simulink model "modello_assex"  (R2021a)
settings: Solver=VariableStepAuto  StartTime=0.0  StopTime=0.2  RelTol=1e-3
InitFcn:
  | global par;
  | 
  | par = parametri();
undefined symbols (not defined in the file or in its folder): accelerazioni
settings Model: Creator=user  LastModifiedBy=stefa
settings SolverCC: AlgebraicLoopSolver=TrustRegion
settings DebuggingCC: SFMachineParentedDataDiag=warning

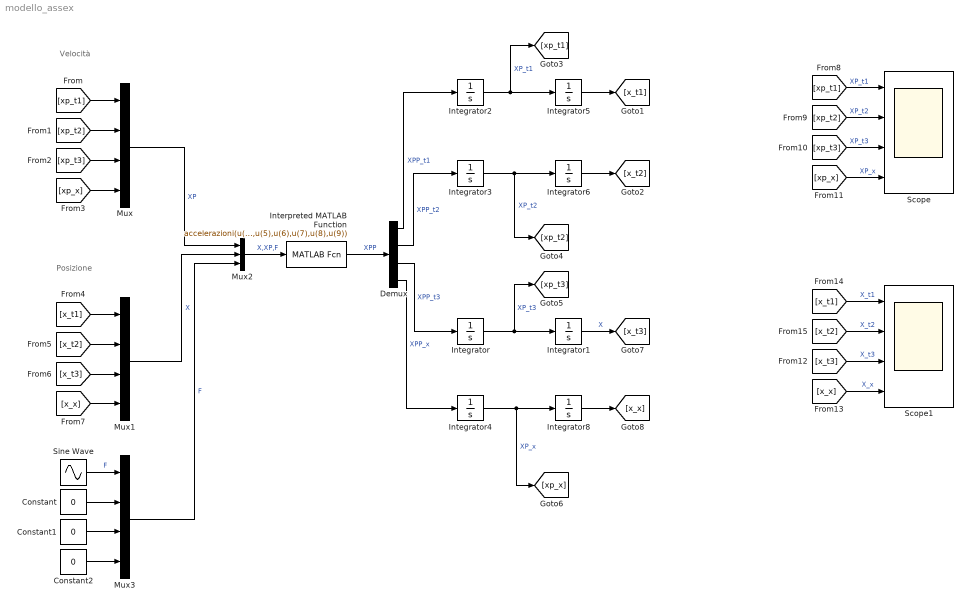
== system modello_assex ==
  note: Posizione
  note: Velocità
  Constant : Constant  Value=0
  Constant1 : Constant  Value=0
  Constant2 : Constant  Value=0
  Demux : Demux
  Integrator{,2..4} (4 alike) : Integrator
  Integrator1 : Integrator  InitialCondition=par.V(3,par.i)
  Integrator5 : Integrator  InitialCondition=par.V(1,par.i)
  Integrator6 : Integrator  InitialCondition=par.V(2,par.i)
  Integrator8 : Integrator  InitialCondition=par.V(4,par.i)
  Interpreted MATLAB Function : MATLABFcn  MATLABFcn=accelerazioni(u(1),u(2),u(3),u(4),u(5),u(6),u(7),u(8),u(9))  OutputDimensions=4
  Mux : Mux
  Mux1 : Mux
  Mux2 : Mux  Inputs=3
  Mux3 : Mux
  Scope : Scope  NumInputPorts=4
  Scope1 : Scope  NumInputPorts=4
  Sine Wave : Sin  Amplitude=0  Frequency=600  SampleTime=0
  wires:
  Interpreted MATLAB Function/1 -> Demux/1  "XPP"
  [xp_t1] -> Mux/1
  [xp_t2] -> Mux/2
  [xp_t3] -> Mux/3
  [xp_x] -> Mux/4
  [x_t3] -> Mux1/3
  [x_t1] -> Mux1/1
  [x_t2] -> Mux1/2
  [x_x] -> Mux1/4
  Mux2/1 -> Interpreted MATLAB Function/1  "X,XP,F"
  Mux/1 -> Mux2/1  "XP"
  Mux1/1 -> Mux2/2  "X"
  [xp_x] -> Scope/4  "XP_x"
  [xp_t3] -> Scope/3  "XP_t3"
  [xp_t2] -> Scope/2  "XP_t2"
  [xp_t1] -> Scope/1  "XP_t1"
  [x_t2] -> Scope1/2  "X_t2"
  [x_t3] -> Scope1/3  "X_t3"
  [x_x] -> Scope1/4  "X_x"
  [x_t1] -> Scope1/1  "X_t1"
  Demux/1 -> Integrator2/1  "XPP_t1"
  Demux/2 -> Integrator3/1  "XPP_t2"
  Demux/3 -> Integrator/1  "XPP_t3"
  Demux/4 -> Integrator4/1  "XPP_x"
  Integrator2/1 -> [xp_t1], Integrator5/1  "XP_t1"
  Integrator3/1 -> [xp_t2], Integrator6/1  "XP_t2"
  Integrator/1 -> [xp_t3], Integrator1/1  "XP_t3"
  Integrator4/1 -> [xp_x], Integrator8/1  "XP_x"
  Integrator5/1 -> [x_t1]
  Integrator6/1 -> [x_t2]
  Integrator1/1 -> [x_t3]  "X"
  Integrator8/1 -> [x_x]
  Sine Wave/1 -> Mux3/1  "F"
  Constant/1 -> Mux3/2
  Constant1/1 -> Mux3/3
  Constant2/1 -> Mux3/4
  Mux3/1 -> Mux2/3  "F"
